simulink model "Estacion_San_Mateo"  (R2017a)
settings: Solver=VariableStepAuto  StartTime=0.0  StopTime=1440  RelTol=1e-3
libraries: simulink x8
settings Model: Creator=Cesar Cardozo  LastModifiedBy=Cesar Cardozo

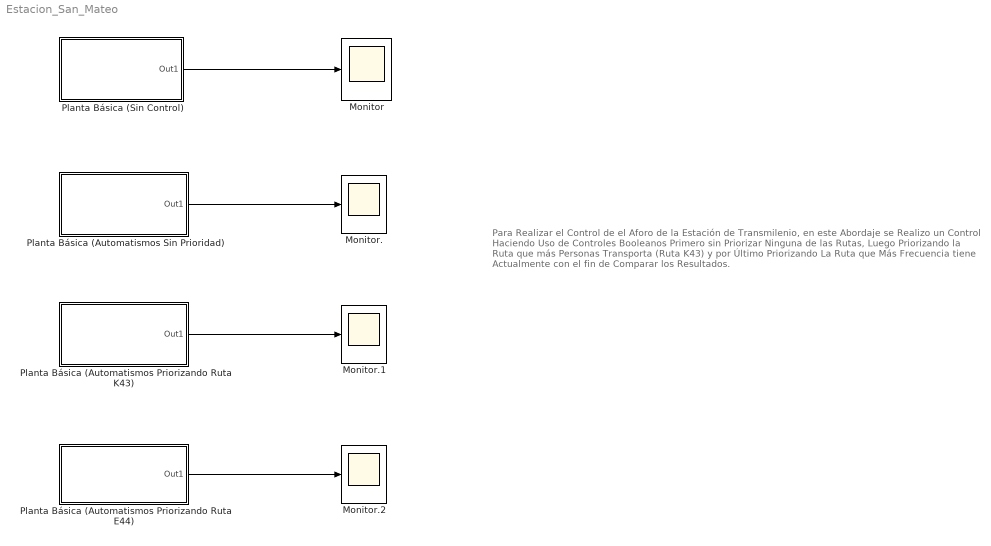
== system Estacion_San_Mateo ==
  note: Para Realizar el Control de el Aforo de la Estación de Transmilenio,
      | en este Abordaje se Realizo un Control Haciendo Uso de Controles Booleanos
      | Primero sin Priorizar Ninguna de las Rutas, Luego Priorizando la Ruta que más
      | Personas Transporta (Ruta K43) y por Último Priorizando La Ruta que Más
      | Frecuencia tiene Actualmente con el fin de Comparar los Resultados.
  Monitor : Scope
  Monitor. : Scope
  Monitor.1 : Scope
  Monitor.2 : Scope
  Planta Básica (Automatismos Priorizando Ruta E44) : Subsystem
  Planta Básica (Automatismos Priorizando Ruta K43) : Subsystem
  Planta Básica (Automatismos Sin Prioridad) : Subsystem
  Planta Básica (Sin Control) : Subsystem
  wires:
  Planta Básica (Sin Control)/1(Out1) -> Monitor/1
  Planta Básica (Automatismos Sin Prioridad)/1(Out1) -> Monitor./1
  Planta Básica (Automatismos Priorizando Ruta K43)/1(Out1) -> Monitor.1/1
  Planta Básica (Automatismos Priorizando Ruta E44)/1(Out1) -> Monitor.2/1

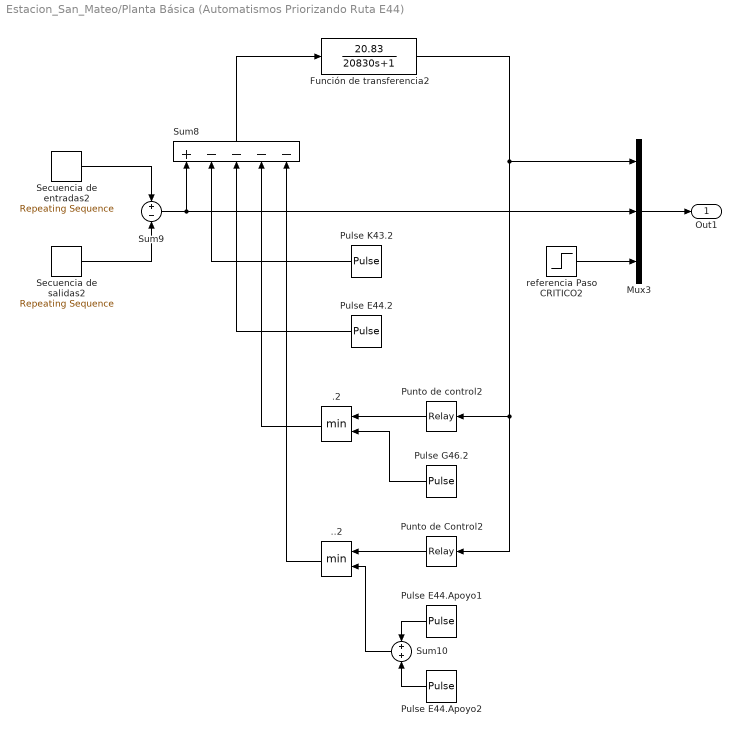
== system Estacion_San_Mateo/Planta Básica (Automatismos Priorizando Ruta E44) ==
  ..2 : MinMax  Inputs=2
  .2 : MinMax  Inputs=2
  Función de transferencia2 : TransferFcn  Numerator=[20.83]  Denominator=[20830 1]
  Mux3 : Mux  Inputs=3
  Pulse E44.2 : DiscretePulseGenerator  PulseType=Time based  Amplitude=3.52  Period=3  PulseWidth=33  PhaseDelay=1
  Pulse E44.Apoyo1 : DiscretePulseGenerator  PulseType=Time based  Amplitude=3.52  Period=2.5  PulseWidth=40  PhaseDelay=2.5
  Pulse E44.Apoyo2 : DiscretePulseGenerator  PulseType=Time based  Amplitude=3.52  Period=2.5  PulseWidth=40  PhaseDelay=2.5
  Pulse G46.2 : DiscretePulseGenerator  PulseType=Time based  Period=5  PulseWidth=20
  Pulse K43.2 : DiscretePulseGenerator  PulseType=Time based  Amplitude=5.2  Period=3  PulseWidth=33
  Punto de Control2 : Relay  OnSwitchValue=50  OffSwitchValue=50  OnOutputValue=100  ZeroCross=off
  Punto de control2 : Relay  OnSwitchValue=50  OffSwitchValue=50  OnOutputValue=0  OffOutputValue=100  ZeroCross=off
  Secuencia de entradas2 : simulink/Sources/Repeating Sequence  rep_seq_t=[0 210 330 540 900 1030 1380 1440]  rep_seq_y=[0 0 500 150 90 180 0 0]
  Secuencia de salidas2 : simulink/Sources/Repeating Sequence  rep_seq_t=[0 270 420 960 1110 1260 1320 1380 1440]  rep_seq_y=[0 0 100 180 400 150 150 0 0]
  Sum10 : Sum
  Sum8 : Sum  Inputs=+----
  Sum9 : Sum  Inputs=+|-
  referencia Paso CRITICO2 : Step  Time=0  After=60  SampleTime=0
  Out1 : Outport
  wires:
  Sum8/1 -> Función de transferencia2/1
  ..2/1 -> Sum8/5
  Secuencia de salidas2/1 -> Sum9/2
  Mux3/1 -> Out1/1
  Punto de control2/1 -> .2/1
  Pulse K43.2/1 -> Sum8/2
  .2/1 -> Sum8/4
  referencia Paso CRITICO2/1 -> Mux3/3
  Sum9/1 -> Sum8/1, Mux3/2
  Secuencia de entradas2/1 -> Sum9/1
  Pulse E44.Apoyo1/1 -> Sum10/1
  Pulse E44.Apoyo2/1 -> Sum10/2
  Pulse G46.2/1 -> .2/2
  Función de transferencia2/1 -> Mux3/1, Punto de control2/1, Punto de Control2/1
  Punto de Control2/1 -> ..2/1
  Sum10/1 -> ..2/2
  Pulse E44.2/1 -> Sum8/3

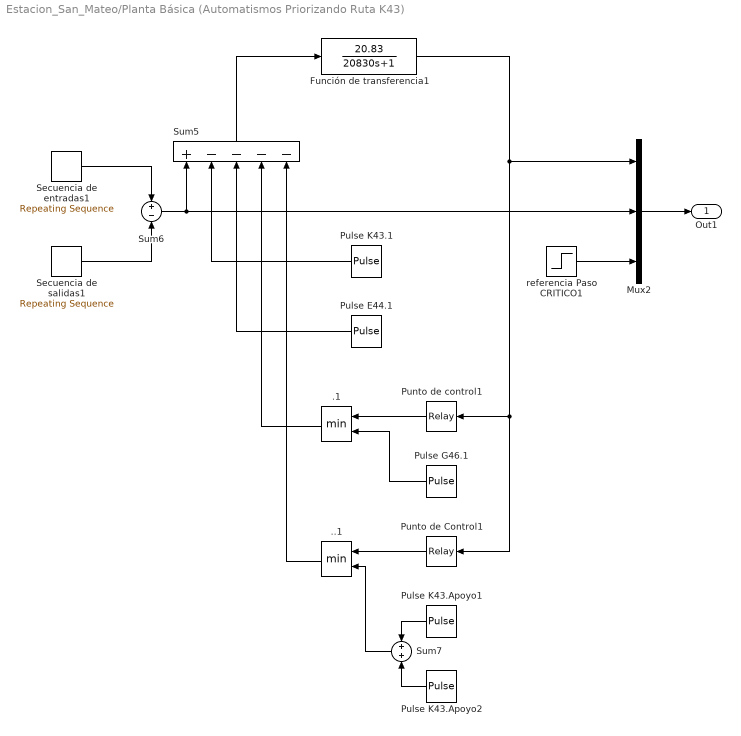
== system Estacion_San_Mateo/Planta Básica (Automatismos Priorizando Ruta K43) ==
  ..1 : MinMax  Inputs=2
  .1 : MinMax  Inputs=2
  Función de transferencia1 : TransferFcn  Numerator=[20.83]  Denominator=[20830 1]
  Mux2 : Mux  Inputs=3
  Pulse E44.1 : DiscretePulseGenerator  PulseType=Time based  Amplitude=3.52  Period=3  PulseWidth=33  PhaseDelay=1
  Pulse G46.1 : DiscretePulseGenerator  PulseType=Time based  Period=5  PulseWidth=20
  Pulse K43.1 : DiscretePulseGenerator  PulseType=Time based  Amplitude=5.2  Period=3  PulseWidth=33
  Pulse K43.Apoyo1 : DiscretePulseGenerator  PulseType=Time based  Amplitude=5.2  Period=2.5  PulseWidth=40
  Pulse K43.Apoyo2 : DiscretePulseGenerator  PulseType=Time based  Amplitude=5.2  Period=2.5  PulseWidth=40
  Punto de Control1 : Relay  OnSwitchValue=50  OffSwitchValue=50  OnOutputValue=100  ZeroCross=off
  Punto de control1 : Relay  OnSwitchValue=50  OffSwitchValue=50  OnOutputValue=0  OffOutputValue=100  ZeroCross=off
  Secuencia de entradas1 : simulink/Sources/Repeating Sequence  rep_seq_t=[0 210 330 540 900 1030 1380 1440]  rep_seq_y=[0 0 500 150 90 180 0 0]
  Secuencia de salidas1 : simulink/Sources/Repeating Sequence  rep_seq_t=[0 270 420 960 1110 1260 1320 1380 1440]  rep_seq_y=[0 0 100 180 400 150 150 0 0]
  Sum5 : Sum  Inputs=+----
  Sum6 : Sum  Inputs=+|-
  Sum7 : Sum
  referencia Paso CRITICO1 : Step  Time=0  After=60  SampleTime=0
  Out1 : Outport
  wires:
  Sum5/1 -> Función de transferencia1/1
  Función de transferencia1/1 -> Punto de Control1/1, Punto de control1/1, Mux2/1
  ..1/1 -> Sum5/5
  Pulse K43.1/1 -> Sum5/2
  referencia Paso CRITICO1/1 -> Mux2/3
  Secuencia de salidas1/1 -> Sum6/2
  Pulse E44.1/1 -> Sum5/3
  .1/1 -> Sum5/4
  Mux2/1 -> Out1/1
  Pulse K43.Apoyo1/1 -> Sum7/1
  Punto de control1/1 -> .1/1
  Sum7/1 -> ..1/2
  Secuencia de entradas1/1 -> Sum6/1
  Punto de Control1/1 -> ..1/1
  Sum6/1 -> Mux2/2, Sum5/1
  Pulse G46.1/1 -> .1/2
  Pulse K43.Apoyo2/1 -> Sum7/2

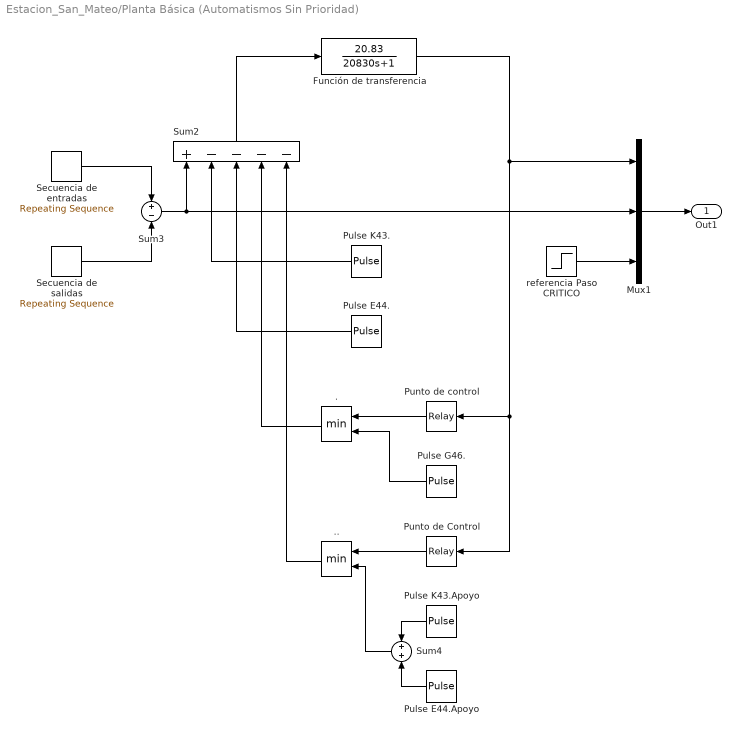
== system Estacion_San_Mateo/Planta Básica (Automatismos Sin Prioridad) ==
  . : MinMax  Inputs=2
  .. : MinMax  Inputs=2
  Función de transferencia : TransferFcn  Numerator=[20.83]  Denominator=[20830 1]
  Mux1 : Mux  Inputs=3
  Pulse E44. : DiscretePulseGenerator  PulseType=Time based  Amplitude=3.52  Period=3  PulseWidth=33  PhaseDelay=1
  Pulse E44.Apoyo : DiscretePulseGenerator  PulseType=Time based  Amplitude=3.52  Period=2.5  PulseWidth=40  PhaseDelay=2.5
  Pulse G46. : DiscretePulseGenerator  PulseType=Time based  Period=5  PulseWidth=20
  Pulse K43. : DiscretePulseGenerator  PulseType=Time based  Amplitude=5.2  Period=3  PulseWidth=33
  Pulse K43.Apoyo : DiscretePulseGenerator  PulseType=Time based  Amplitude=5.2  Period=2.5  PulseWidth=40
  Punto de Control : Relay  OnSwitchValue=50  OffSwitchValue=50  OnOutputValue=100  ZeroCross=off
  Punto de control : Relay  OnSwitchValue=50  OffSwitchValue=50  OnOutputValue=0  OffOutputValue=100  ZeroCross=off
  Secuencia de entradas : simulink/Sources/Repeating Sequence  rep_seq_t=[0 210 330 540 900 1030 1380 1440]  rep_seq_y=[0 0 500 150 90 180 0 0]
  Secuencia de salidas : simulink/Sources/Repeating Sequence  rep_seq_t=[0 270 420 960 1110 1260 1320 1380 1440]  rep_seq_y=[0 0 100 180 400 150 150 0 0]
  Sum2 : Sum  Inputs=+----
  Sum3 : Sum  Inputs=+|-
  Sum4 : Sum
  referencia Paso CRITICO : Step  Time=0  After=60  SampleTime=0
  Out1 : Outport
  wires:
  Sum2/1 -> Función de transferencia/1
  Mux1/1 -> Out1/1
  Pulse K43./1 -> Sum2/2
  Sum3/1 -> Mux1/2, Sum2/1
  Pulse E44./1 -> Sum2/3
  Pulse G46./1 -> ./2
  Punto de control/1 -> ./1
  Pulse K43.Apoyo/1 -> Sum4/1
  Pulse E44.Apoyo/1 -> Sum4/2
  Punto de Control/1 -> ../1
  ./1 -> Sum2/4
  ../1 -> Sum2/5
  Secuencia de salidas/1 -> Sum3/2
  Sum4/1 -> ../2
  Secuencia de entradas/1 -> Sum3/1
  referencia Paso CRITICO/1 -> Mux1/3
  Función de transferencia/1 -> Punto de Control/1, Punto de control/1, Mux1/1

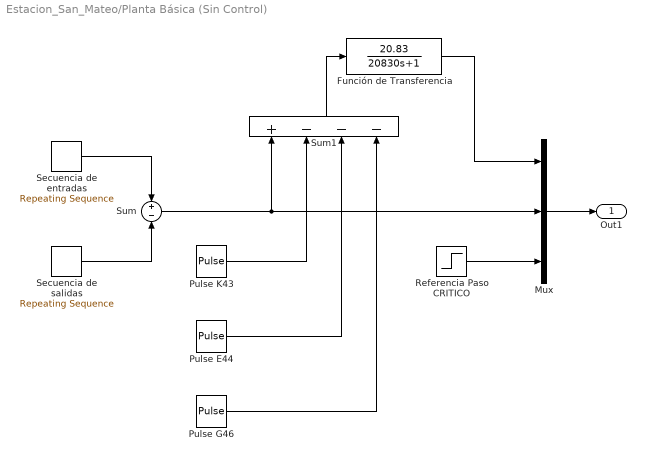
== system Estacion_San_Mateo/Planta Básica (Sin Control) ==
  Función de Transferencia : TransferFcn  Numerator=[20.83]  Denominator=[20830 1]
  Mux : Mux  Inputs=3
  Pulse E44 : DiscretePulseGenerator  PulseType=Time based  Amplitude=3.52  Period=3  PulseWidth=33  PhaseDelay=1
  Pulse G46 : DiscretePulseGenerator  PulseType=Time based  Period=5  PulseWidth=20
  Pulse K43 : DiscretePulseGenerator  PulseType=Time based  Amplitude=5.2  Period=3  PulseWidth=33  VectorParams1D=off
  Referencia Paso CRITICO : Step  Time=0  After=60  SampleTime=0
  "Secuencia de salidas " : simulink/Sources/Repeating Sequence  rep_seq_t=[0 270 420 960 1110 1260 1320 1380 1440]  rep_seq_y=[0 0 100 180 400 150 150 0 0]
  Secuencia de entradas : simulink/Sources/Repeating Sequence  rep_seq_t=[0 210 330 540 900 1030 1380 1440]  rep_seq_y=[0 0 500 150 90 180 0 0]
  Sum : Sum  Inputs=+|-
  Sum1 : Sum  Inputs=+---
  Out1 : Outport
  wires:
  Sum1/1 -> Función de Transferencia/1
  Mux/1 -> Out1/1
  Función de Transferencia/1 -> Mux/1
  Pulse G46/1 -> Sum1/4
  Sum/1 -> Mux/2, Sum1/1
  Secuencia de entradas/1 -> Sum/1
  "Secuencia de salidas "/1 -> Sum/2
  Pulse E44/1 -> Sum1/3
  Referencia Paso CRITICO/1 -> Mux/3
  Pulse K43/1 -> Sum1/2
